simulink model "HITL_HEXA_MISSION"  (R2023b)
settings: Solver=FixedStepDiscrete  StartTime=0.0  StopTime=inf  FixedStep=1/250  RelTol=1e-3  EnableMultiTasking=on
values from neighbouring files (symbols this model uses):
  SampleTime = 1/250    (= 0.004)    [Init_FLIGHT_Hexacopter.m]    (also in Init_FLIGHT_Hexacopter_fromNCMS.m = 0.01)
undefined symbols (not defined in the file or in its folder): control, IDLEPWM, MC_PITCH_P, MC_PITCHRATE_D, MC_PITCHRATE_I, MC_PITCHRATE_P, MC_ROLL_P, MC_ROLLRATE_D, MC_ROLLRATE_I, MC_ROLLRATE_P, MC_YAW_P, MC_YAWRATE_D, MC_YAWRATE_I, MC_YAWRATE_P, MPC_XY_P, MPC_XY_VEL_MAX, MPC_Z_D, MPC_Z_I, MPC_Z_P, MPC_Z_VEL_D_ACC, MPC_Z_VEL_I_ACC, MPC_Z_VEL_MAX_DN, MPC_Z_VEL_MAX_UP, MPC_Z_VEL_P_ACC, noutputs, output, pitch, pitch_body, roll, roll_body, TargetHardware, thrust_body, timestamp, x, y, yaw, yaw_body, z
libraries: px4lib x45, px4uORBlib x19, slpidlib x10, simulink x9, px4Utilslib x5, simulink_extras x5, uavalgslib x3, px4Sensorslib x2, sharedutil x1, sharedtransform x1
(part 2 of 4)

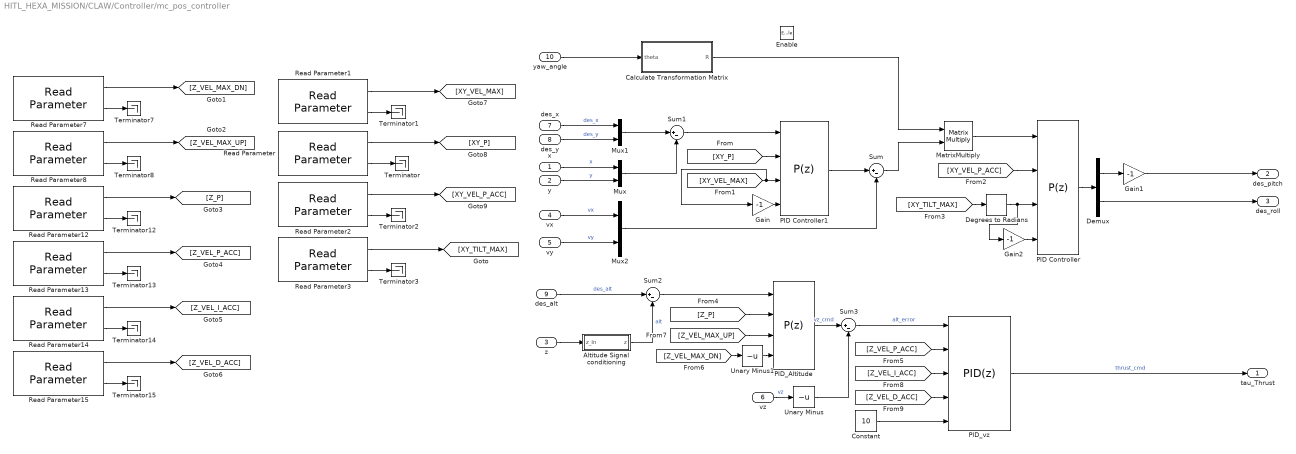
== system HITL_HEXA_MISSION/CLAW/Controller/mc_pos_controller ==
  x : Inport
  y : Inport  Port=2
  z : Inport  Port=3
  vx : Inport  Port=4
  vy : Inport  Port=5
  vz : Inport  Port=6
  des_x : Inport  Port=7
  des_y : Inport  Port=8
  des_alt : Inport  Port=9
  yaw_angle : Inport  Port=10
  Enable : EnablePort
  Altitude Signal conditioning : Subsystem
  Calculate Transformation Matrix : Subsystem
  Constant : Constant  Value=10
  Degrees to Radians : simulink_extras/Transformations/Degrees to Radians
  Demux : Demux  Outputs=2
  Gain : Gain  Gain=-1
  Gain1 : Gain  Gain=-1
  Gain2 : Gain  Gain=-1
  MatrixMultiply : Product  Multiplication=Matrix(*)
  Mux : Mux  Inputs=2
  Mux1 : Mux  Inputs=2
  Mux2 : Mux  Inputs=2
  PID Controller : slpidlib/PID Controller  Controller=P  Form=Parallel  TimeDomain=Discrete-time  UseExternalTs=off  SampleTime=-1  IntegratorMethod=Forward Euler  FilterMethod=Forward Euler  ControllerParametersSource=external  P=0.3  I=0  UseKiTs=off  D=0  N=20  UseFilter=on  TunerSelectOption=Transfer Function Based (PID Tuner App)  InitialConditionSource=internal  InitialConditionForIntegrator=0  InitialConditionForFilter=0  DifferentiatorICPrevScaledInput=0  ExternalReset=none  TrackingMode=off  Kt=1  LimitOutput=on  SatLimitsSource=external  UpperSaturationLimit=20*pi/180  LowerSaturationLimit=-20*pi/180  LinearizeAsGain=on  AntiWindupMode=clamping  Kb=1  LimitIntegrator=off  UpperIntegratorSaturationLimit=inf  LowerIntegratorSaturationLimit=-inf  POutMin=[]  POutMax=[]  IOutMin=[]  IOutMax=[]  DOutMin=[]  DOutMax=[]  NOutMin=[]  NOutMax=[]  SumOutMin=[]  SumOutMax=[]  SaturationOutMin=[]  SaturationOutMax=[]  PParamMin=[]  PParamMax=[]  IParamMin=[]  IParamMax=[]  DParamMin=[]  DParamMax=[]  NParamMin=[]  NParamMax=[]  KbParamMin=[]  KbParamMax=[]  KtParamMin=[]  KtParamMax=[]  KbOutMin=[]  KbOutMax=[]  KtOutMin=[]  KtOutMax=[]  IntegratorOutMin=[]  IntegratorOutMax=[]  FilterOutMin=[]  FilterOutMax=[]  SumI1OutMin=[]  SumI1OutMax=[]  SumI2OutMin=[]  SumI2OutMax=[]  SumI3OutMin=[]  SumI3OutMax=[]  SumI4OutMin=[]  SumI4OutMax=[]  SumDOutMin=[]  SumDOutMax=[]  DifferentiatorOutMin=[]  DifferentiatorOutMax=[]  FilterDiffOutCoefMin=[]  FilterDiffOutCoefMax=[]  ReciprocalOutMin=[]  ReciprocalOutMax=[]  SumDenOutMin=[]  SumDenOutMax=[]  SumNumOutMin=[]  SumNumOutMax=[]  DivideOutMin=[]  DivideOutMax=[]  UdiffTsProdOutMin=[]  UdiffTsProdOutMax=[]  NTsProdOutMin=[]  NTsProdOutMax=[]  UintegralTsProdOutMin=[]  UintegralTsProdOutMax=[]  UngainTsProdOutMin=[]  UngainTsProdOutMax=[]  ClampingZeroOutDataTypeStr=Inherit: Inherit via back propagation  ClampingZeroOutMin=[]  ClampingZeroOutMax=[]  FilterDenConstantOutDataTypeStr=Inherit: Inherit via back propagation  FilterDenConstantOutMin=[]  FilterDenConstantOutMax=[]  PCopyOutDataTypeStr=Inherit: Inherit via back propagation  PCopyOutMin=[]  PCopyOutMax=[]  NCopyOutDataTypeStr=Inherit: Inherit via back propagation  NCopyOutMin=[]  NCopyOutMax=[]  IntegratorContinuousStateAttributes=''  IntegratorStateMustResolveToSignalObject=off  IntegratorRTWStateStorageClass=Auto  FilterContinuousStateAttributes=''  FilterStateMustResolveToSignalObject=off  FilterRTWStateStorageClass=Auto  ParallelPVariant=ExternalParameters  IdealPVariant=Disabled  IVariant=Disabled  DVariant=Disabled  IntegratorVariant=Disabled  SatVariant=External  AWVariant=Disabled  PCopyVariant=Disabled  TRVariant=Disabled  FdbkBlocksVariant=Forward  IdealPFdbkVariant=Disabled  SatFdbkVariant=Disabled  DerivativeFilterVariant=Disabled  NVariant=Disabled  NCopyVariant=Disabled_SignalSpec  FilterICVariant=Disabled  IntegratorICVariant=Disabled  ExternalResetVariant=Disabled  TRSumVariant=Passthrough  SumFdbkVariant=Disabled  SumVariant=Passthrough_P  TsampFilterVariant=InternalTs  TsampNgainVariant=Passthrough  TsampIntegralVariant=Disabled_SignalSpec  ExternalSaturationOutDataTypeStr=Inherit: Same as second input
  PID Controller1 : slpidlib/PID Controller  Controller=P  Form=Parallel  TimeDomain=Discrete-time  UseExternalTs=off  SampleTime=-1  IntegratorMethod=Forward Euler  FilterMethod=Forward Euler  ControllerParametersSource=external  P=MPC_XY_P  I=0  UseKiTs=off  D=0  N=20  UseFilter=on  TunerSelectOption=Transfer Function Based (PID Tuner App)  InitialConditionSource=internal  InitialConditionForIntegrator=0  InitialConditionForFilter=0  DifferentiatorICPrevScaledInput=0  ExternalReset=none  TrackingMode=off  Kt=1  LimitOutput=on  SatLimitsSource=external  UpperSaturationLimit=abs(MPC_XY_VEL_MAX)  LowerSaturationLimit=-abs(MPC_XY_VEL_MAX)  LinearizeAsGain=on  AntiWindupMode=clamping  Kb=1  LimitIntegrator=off  UpperIntegratorSaturationLimit=inf  LowerIntegratorSaturationLimit=-inf  POutMin=[]  POutMax=[]  IOutMin=[]  IOutMax=[]  DOutMin=[]  DOutMax=[]  NOutMin=[]  NOutMax=[]  SumOutMin=[]  SumOutMax=[]  SaturationOutMin=[]  SaturationOutMax=[]  PParamMin=[]  PParamMax=[]  IParamMin=[]  IParamMax=[]  DParamMin=[]  DParamMax=[]  NParamMin=[]  NParamMax=[]  KbParamMin=[]  KbParamMax=[]  KtParamMin=[]  KtParamMax=[]  KbOutMin=[]  KbOutMax=[]  KtOutMin=[]  KtOutMax=[]  IntegratorOutMin=[]  IntegratorOutMax=[]  FilterOutMin=[]  FilterOutMax=[]  SumI1OutMin=[]  SumI1OutMax=[]  SumI2OutMin=[]  SumI2OutMax=[]  SumI3OutMin=[]  SumI3OutMax=[]  SumI4OutMin=[]  SumI4OutMax=[]  SumDOutMin=[]  SumDOutMax=[]  DifferentiatorOutMin=[]  DifferentiatorOutMax=[]  FilterDiffOutCoefMin=[]  FilterDiffOutCoefMax=[]  ReciprocalOutMin=[]  ReciprocalOutMax=[]  SumDenOutMin=[]  SumDenOutMax=[]  SumNumOutMin=[]  SumNumOutMax=[]  DivideOutMin=[]  DivideOutMax=[]  UdiffTsProdOutMin=[]  UdiffTsProdOutMax=[]  NTsProdOutMin=[]  NTsProdOutMax=[]  UintegralTsProdOutMin=[]  UintegralTsProdOutMax=[]  UngainTsProdOutMin=[]  UngainTsProdOutMax=[]  ClampingZeroOutDataTypeStr=Inherit: Inherit via back propagation  ClampingZeroOutMin=[]  ClampingZeroOutMax=[]  FilterDenConstantOutDataTypeStr=Inherit: Inherit via back propagation  FilterDenConstantOutMin=[]  FilterDenConstantOutMax=[]  PCopyOutDataTypeStr=Inherit: Inherit via back propagation  PCopyOutMin=[]  PCopyOutMax=[]  NCopyOutDataTypeStr=Inherit: Inherit via back propagation  NCopyOutMin=[]  NCopyOutMax=[]  IntegratorContinuousStateAttributes=''  IntegratorStateMustResolveToSignalObject=off  IntegratorRTWStateStorageClass=Auto  FilterContinuousStateAttributes=''  FilterStateMustResolveToSignalObject=off  FilterRTWStateStorageClass=Auto  ParallelPVariant=ExternalParameters  IdealPVariant=Disabled  IVariant=Disabled  DVariant=Disabled  IntegratorVariant=Disabled  SatVariant=External  AWVariant=Disabled  PCopyVariant=Disabled  TRVariant=Disabled  FdbkBlocksVariant=Forward  IdealPFdbkVariant=Disabled  SatFdbkVariant=Disabled  DerivativeFilterVariant=Disabled  NVariant=Disabled  NCopyVariant=Disabled_SignalSpec  FilterICVariant=Disabled  IntegratorICVariant=Disabled  ExternalResetVariant=Disabled  TRSumVariant=Passthrough  SumFdbkVariant=Disabled  SumVariant=Passthrough_P  TsampFilterVariant=InternalTs  TsampNgainVariant=Passthrough  TsampIntegralVariant=Disabled_SignalSpec  ExternalSaturationOutDataTypeStr=Inherit: Same as second input
  PID_Altitude : slpidlib/PID Controller  Controller=P  Form=Parallel  TimeDomain=Discrete-time  UseExternalTs=off  SampleTime=-1  IntegratorMethod=Backward Euler  FilterMethod=Forward Euler  ControllerParametersSource=external  P=MPC_Z_P  I=MPC_Z_I  UseKiTs=off  D=MPC_Z_D  N=10  UseFilter=on  TunerSelectOption=Transfer Function Based (PID Tuner App)  InitialConditionSource=internal  InitialConditionForIntegrator=0  InitialConditionForFilter=0  DifferentiatorICPrevScaledInput=0  ExternalReset=none  TrackingMode=off  Kt=1  LimitOutput=on  SatLimitsSource=external  UpperSaturationLimit=MPC_Z_VEL_MAX_UP  LowerSaturationLimit=-abs(MPC_Z_VEL_MAX_DN)  LinearizeAsGain=off  AntiWindupMode=clamping  Kb=1  LimitIntegrator=off  UpperIntegratorSaturationLimit=inf  LowerIntegratorSaturationLimit=-inf  POutMin=[]  POutMax=[]  IOutMin=[]  IOutMax=[]  DOutMin=[]  DOutMax=[]  NOutMin=[]  NOutMax=[]  SumOutMin=[]  SumOutMax=[]  SaturationOutMin=[]  SaturationOutMax=[]  PParamMin=[]  PParamMax=[]  IParamMin=[]  IParamMax=[]  DParamMin=[]  DParamMax=[]  NParamMin=[]  NParamMax=[]  KbParamMin=[]  KbParamMax=[]  KtParamMin=[]  KtParamMax=[]  KbOutMin=[]  KbOutMax=[]  KtOutMin=[]  KtOutMax=[]  IntegratorOutMin=[]  IntegratorOutMax=[]  FilterOutMin=[]  FilterOutMax=[]  SumI1OutMin=[]  SumI1OutMax=[]  SumI2OutMin=[]  SumI2OutMax=[]  SumI3OutMin=[]  SumI3OutMax=[]  SumI4OutMin=[]  SumI4OutMax=[]  SumDOutMin=[]  SumDOutMax=[]  DifferentiatorOutMin=[]  DifferentiatorOutMax=[]  FilterDiffOutCoefMin=[]  FilterDiffOutCoefMax=[]  ReciprocalOutMin=[]  ReciprocalOutMax=[]  SumDenOutMin=[]  SumDenOutMax=[]  SumNumOutMin=[]  SumNumOutMax=[]  DivideOutMin=[]  DivideOutMax=[]  UdiffTsProdOutMin=[]  UdiffTsProdOutMax=[]  NTsProdOutMin=[]  NTsProdOutMax=[]  UintegralTsProdOutMin=[]  UintegralTsProdOutMax=[]  UngainTsProdOutMin=[]  UngainTsProdOutMax=[]  ClampingZeroOutDataTypeStr=Inherit: Inherit via back propagation  ClampingZeroOutMin=[]  ClampingZeroOutMax=[]  FilterDenConstantOutDataTypeStr=Inherit: Inherit via back propagation  FilterDenConstantOutMin=[]  FilterDenConstantOutMax=[]  PCopyOutDataTypeStr=Inherit: Inherit via back propagation  PCopyOutMin=[]  PCopyOutMax=[]  NCopyOutDataTypeStr=Inherit: Inherit via back propagation  NCopyOutMin=[]  NCopyOutMax=[]  IntegratorContinuousStateAttributes=''  IntegratorStateMustResolveToSignalObject=off  IntegratorRTWStateStorageClass=Auto  FilterContinuousStateAttributes=''  FilterStateMustResolveToSignalObject=off  FilterRTWStateStorageClass=Auto  ParallelPVariant=ExternalParameters  IdealPVariant=Disabled  IVariant=Disabled  DVariant=Disabled  IntegratorVariant=Disabled  SatVariant=External  AWVariant=Disabled  PCopyVariant=Disabled  TRVariant=Disabled  FdbkBlocksVariant=Forward  IdealPFdbkVariant=Disabled  SatFdbkVariant=Disabled  DerivativeFilterVariant=Disabled  NVariant=Disabled  NCopyVariant=Disabled_SignalSpec  FilterICVariant=Disabled  IntegratorICVariant=Disabled  ExternalResetVariant=Disabled  TRSumVariant=Passthrough  SumFdbkVariant=Disabled  SumVariant=Passthrough_P  TsampFilterVariant=InternalTs  TsampNgainVariant=Passthrough  TsampIntegralVariant=Disabled_SignalSpec  ExternalSaturationOutDataTypeStr=Inherit: Same as second input
  PID_vz : slpidlib/PID Controller  Controller=PID  Form=Parallel  TimeDomain=Discrete-time  UseExternalTs=off  SampleTime=-1  IntegratorMethod=Backward Euler  FilterMethod=Forward Euler  ControllerParametersSource=external  P=MPC_Z_VEL_P_ACC  I=MPC_Z_VEL_I_ACC  UseKiTs=off  D=MPC_Z_VEL_D_ACC  N=10  UseFilter=on  TunerSelectOption=Transfer Function Based (PID Tuner App)  InitialConditionSource=internal  InitialConditionForIntegrator=0  InitialConditionForFilter=0  DifferentiatorICPrevScaledInput=0  ExternalReset=none  TrackingMode=off  Kt=1  LimitOutput=on  SatLimitsSource=internal  UpperSaturationLimit=1  LowerSaturationLimit=0  LinearizeAsGain=off  AntiWindupMode=clamping  Kb=1  LimitIntegrator=off  UpperIntegratorSaturationLimit=inf  LowerIntegratorSaturationLimit=-inf  POutMin=[]  POutMax=[]  IOutMin=[]  IOutMax=[]  DOutMin=[]  DOutMax=[]  NOutMin=[]  NOutMax=[]  SumOutMin=[]  SumOutMax=[]  SaturationOutMin=[]  SaturationOutMax=[]  PParamMin=[]  PParamMax=[]  IParamMin=[]  IParamMax=[]  DParamMin=[]  DParamMax=[]  NParamMin=[]  NParamMax=[]  KbParamMin=[]  KbParamMax=[]  KtParamMin=[]  KtParamMax=[]  KbOutMin=[]  KbOutMax=[]  KtOutMin=[]  KtOutMax=[]  IntegratorOutMin=[]  IntegratorOutMax=[]  FilterOutMin=[]  FilterOutMax=[]  SumI1OutMin=[]  SumI1OutMax=[]  SumI2OutMin=[]  SumI2OutMax=[]  SumI3OutMin=[]  SumI3OutMax=[]  SumI4OutMin=[]  SumI4OutMax=[]  SumDOutMin=[]  SumDOutMax=[]  DifferentiatorOutMin=[]  DifferentiatorOutMax=[]  FilterDiffOutCoefMin=[]  FilterDiffOutCoefMax=[]  ReciprocalOutMin=[]  ReciprocalOutMax=[]  SumDenOutMin=[]  SumDenOutMax=[]  SumNumOutMin=[]  SumNumOutMax=[]  DivideOutMin=[]  DivideOutMax=[]  UdiffTsProdOutMin=[]  UdiffTsProdOutMax=[]  NTsProdOutMin=[]  NTsProdOutMax=[]  UintegralTsProdOutMin=[]  UintegralTsProdOutMax=[]  UngainTsProdOutMin=[]  UngainTsProdOutMax=[]  ClampingZeroOutDataTypeStr=Inherit: Inherit via back propagation  ClampingZeroOutMin=[]  ClampingZeroOutMax=[]  FilterDenConstantOutDataTypeStr=Inherit: Inherit via back propagation  FilterDenConstantOutMin=[]  FilterDenConstantOutMax=[]  PCopyOutDataTypeStr=Inherit: Inherit via back propagation  PCopyOutMin=[]  PCopyOutMax=[]  NCopyOutDataTypeStr=Inherit: Inherit via back propagation  NCopyOutMin=[]  NCopyOutMax=[]  IntegratorContinuousStateAttributes=''  IntegratorStateMustResolveToSignalObject=off  IntegratorRTWStateStorageClass=Auto  FilterContinuousStateAttributes=''  FilterStateMustResolveToSignalObject=off  FilterRTWStateStorageClass=Auto  ParallelPVariant=ExternalParameters  IdealPVariant=Disabled  IVariant=ExternalParameters  DVariant=ExternalParameters  IntegratorVariant=Discrete  SatVariant=Enabled  AWVariant=DiscClampingParallel  PCopyVariant=Disabled  TRVariant=Disabled  FdbkBlocksVariant=Feedback  IdealPFdbkVariant=Passthrough  SatFdbkVariant=Passthrough  DerivativeFilterVariant=ForwardEulerFilter  NVariant=ExternalParameters  NCopyVariant=Disabled  FilterICVariant=InternalICsFilter  IntegratorICVariant=InternalICs  ExternalResetVariant=Disabled  TRSumVariant=Passthrough  SumFdbkVariant=Enabled  SumVariant=Sum_PID  TsampFilterVariant=InternalTs  TsampNgainVariant=Passthrough  TsampIntegralVariant=Disabled_SignalSpec  ExternalSaturationOutDataTypeStr=Inherit: Same as second input
  Read Parameter : px4lib/Read Parameter  ParameterName=SL_XY_P  DataType=FLOAT  SampleTime=-1
  Read Parameter1 : px4lib/Read Parameter  ParameterName=SL_XY_VEL_MAX  DataType=FLOAT  SampleTime=-1
  Read Parameter12 : px4lib/Read Parameter  ParameterName=SL_Z_P  DataType=FLOAT  SampleTime=-1
  Read Parameter13 : px4lib/Read Parameter  ParameterName=SL_Z_VEL_P_ACC  DataType=FLOAT  SampleTime=-1
  Read Parameter14 : px4lib/Read Parameter  ParameterName=SL_Z_VEL_I_ACC  DataType=FLOAT  SampleTime=-1
  Read Parameter15 : px4lib/Read Parameter  ParameterName=SL_Z_VEL_D_ACC  DataType=FLOAT  SampleTime=-1
  Read Parameter2 : px4lib/Read Parameter  ParameterName=SL_XY_VEL_P_ACC  DataType=FLOAT  SampleTime=-1
  Read Parameter3 : px4lib/Read Parameter  ParameterName=SL_XY_TILT_MAX  DataType=FLOAT  SampleTime=-1
  Read Parameter7 : px4lib/Read Parameter  ParameterName=SL_Z_VEL_MAX_DN  DataType=FLOAT  SampleTime=-1
  Read Parameter8 : px4lib/Read Parameter  ParameterName=SL_Z_VEL_MAX_UP  DataType=FLOAT  SampleTime=-1
  Sum{,1..3} (4 alike) : Sum  Inputs=|+-
  Terminator{,1..3,7..8,12..15} (10 alike) : Terminator
  Unary Minus : UnaryMinus
  Unary Minus1 : UnaryMinus
  tau_Thrust : Outport
  des_pitch : Outport  Port=2
  des_roll : Outport  Port=3
  wires:
  des_alt/1 -> Sum2/1  "des_alt"
  Calculate Transformation Matrix/1(R) -> MatrixMultiply/1
  yaw_angle/1 -> Calculate Transformation Matrix/1(theta)
  Altitude Signal conditioning/1(z) -> Sum2/2  "alt"
  PID_Altitude/1 -> Sum3/1  "vz_cmd"
  vz/1 -> Unary Minus/1  "vz"
  PID_vz/1 -> tau_Thrust/1  "thrust_cmd"
  vx/1 -> Mux2/1  "vx"
  vy/1 -> Mux2/2  "vy"
  Sum2/1 -> PID_Altitude/1
  z/1 -> Altitude Signal conditioning/1(z_In)
  PID Controller/1 -> Demux/1
  Demux/1 -> Gain1/1
  x/1 -> Mux/1  "x"
  y/1 -> Mux/2  "y"
  Demux/2 -> des_roll/1
  Sum/1 -> MatrixMultiply/2
  Mux/1 -> Sum1/2
  Sum1/1 -> PID Controller1/1
  Unary Minus/1 -> Sum3/2
  Sum3/1 -> PID_vz/1  "alt_error"
  des_x/1 -> Mux1/1  "des_x"
  des_y/1 -> Mux1/2  "des_y"
  MatrixMultiply/1 -> PID Controller/1
  PID Controller1/1 -> Sum/1
  Mux1/1 -> Sum1/1
  Gain1/1 -> des_pitch/1
  Mux2/1 -> Sum/2
  Read Parameter14/2 -> Terminator14/1
  Read Parameter12/2 -> Terminator12/1
  Read Parameter14/1 -> [Z_VEL_I_ACC]
  Read Parameter/1 -> [XY_P]
  Read Parameter13/1 -> [Z_VEL_P_ACC]
  Read Parameter8/1 -> [Z_VEL_MAX_UP]
  Read Parameter3/2 -> Terminator3/1
  Read Parameter12/1 -> [Z_P]
  Read Parameter8/2 -> Terminator8/1
  Read Parameter7/2 -> Terminator7/1
  Read Parameter1/1 -> [XY_VEL_MAX]
  Read Parameter2/1 -> [XY_VEL_P_ACC]
  Read Parameter2/2 -> Terminator2/1
  Read Parameter15/1 -> [Z_VEL_D_ACC]
  Read Parameter1/2 -> Terminator1/1
  Read Parameter3/1 -> [XY_TILT_MAX]
  Read Parameter13/2 -> Terminator13/1
  Read Parameter/2 -> Terminator/1
  Read Parameter15/2 -> Terminator15/1
  [XY_P] -> PID Controller1/2
  [XY_VEL_MAX] -> PID Controller1/3, Gain/1
  Gain/1 -> PID Controller1/4
  [XY_VEL_P_ACC] -> PID Controller/2
  [XY_TILT_MAX] -> Degrees to Radians/1
  Degrees to Radians/1 -> Gain2/1, PID Controller/3
  Gain2/1 -> PID Controller/4
  Read Parameter7/1 -> [Z_VEL_MAX_DN]
  [Z_P] -> PID_Altitude/2
  [Z_VEL_MAX_UP] -> PID_Altitude/3
  [Z_VEL_P_ACC] -> PID_vz/2
  [Z_VEL_I_ACC] -> PID_vz/3
  [Z_VEL_D_ACC] -> PID_vz/4
  Constant/1 -> PID_vz/5
  [Z_VEL_MAX_DN] -> Unary Minus1/1
  Unary Minus1/1 -> PID_Altitude/4

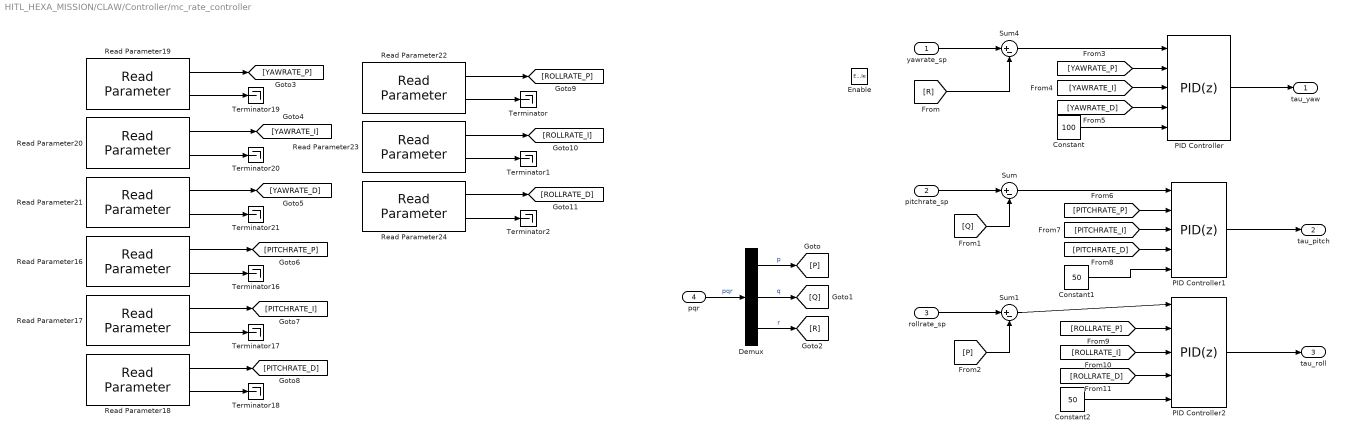
== system HITL_HEXA_MISSION/CLAW/Controller/mc_rate_controller ==
  yawrate_sp : Inport
  pitchrate_sp : Inport  Port=2
  rollrate_sp : Inport  Port=3
  pqr : Inport  Port=4
  Enable : EnablePort
  Constant : Constant  Value=100
  Constant1 : Constant  Value=50
  Constant2 : Constant  Value=50
  Demux : Demux  Outputs=3
  PID Controller : slpidlib/PID Controller  Controller=PID  Form=Parallel  TimeDomain=Discrete-time  UseExternalTs=off  SampleTime=-1  IntegratorMethod=Forward Euler  FilterMethod=Forward Euler  ControllerParametersSource=external  P=MC_YAWRATE_P  I=MC_YAWRATE_I  UseKiTs=off  D=MC_YAWRATE_D  N=100  UseFilter=on  TunerSelectOption=Transfer Function Based (PID Tuner App)  InitialConditionSource=internal  InitialConditionForIntegrator=0  InitialConditionForFilter=0  DifferentiatorICPrevScaledInput=0  ExternalReset=none  TrackingMode=off  Kt=1  LimitOutput=on  SatLimitsSource=internal  UpperSaturationLimit=0.1  LowerSaturationLimit=-0.1  LinearizeAsGain=on  AntiWindupMode=clamping  Kb=1  LimitIntegrator=off  UpperIntegratorSaturationLimit=inf  LowerIntegratorSaturationLimit=-inf  POutMin=[]  POutMax=[]  IOutMin=[]  IOutMax=[]  DOutMin=[]  DOutMax=[]  NOutMin=[]  NOutMax=[]  SumOutMin=[]  SumOutMax=[]  SaturationOutMin=[]  SaturationOutMax=[]  PParamMin=[]  PParamMax=[]  IParamMin=[]  IParamMax=[]  DParamMin=[]  DParamMax=[]  NParamMin=[]  NParamMax=[]  KbParamMin=[]  KbParamMax=[]  KtParamMin=[]  KtParamMax=[]  KbOutMin=[]  KbOutMax=[]  KtOutMin=[]  KtOutMax=[]  IntegratorOutMin=[]  IntegratorOutMax=[]  FilterOutMin=[]  FilterOutMax=[]  SumI1OutMin=[]  SumI1OutMax=[]  SumI2OutMin=[]  SumI2OutMax=[]  SumI3OutMin=[]  SumI3OutMax=[]  SumI4OutMin=[]  SumI4OutMax=[]  SumDOutMin=[]  SumDOutMax=[]  DifferentiatorOutMin=[]  DifferentiatorOutMax=[]  FilterDiffOutCoefMin=[]  FilterDiffOutCoefMax=[]  ReciprocalOutMin=[]  ReciprocalOutMax=[]  SumDenOutMin=[]  SumDenOutMax=[]  SumNumOutMin=[]  SumNumOutMax=[]  DivideOutMin=[]  DivideOutMax=[]  UdiffTsProdOutMin=[]  UdiffTsProdOutMax=[]  NTsProdOutMin=[]  NTsProdOutMax=[]  UintegralTsProdOutMin=[]  UintegralTsProdOutMax=[]  UngainTsProdOutMin=[]  UngainTsProdOutMax=[]  ClampingZeroOutDataTypeStr=Inherit: Inherit via back propagation  ClampingZeroOutMin=[]  ClampingZeroOutMax=[]  FilterDenConstantOutDataTypeStr=Inherit: Inherit via back propagation  FilterDenConstantOutMin=[]  FilterDenConstantOutMax=[]  PCopyOutDataTypeStr=Inherit: Inherit via back propagation  PCopyOutMin=[]  PCopyOutMax=[]  NCopyOutDataTypeStr=Inherit: Inherit via back propagation  NCopyOutMin=[]  NCopyOutMax=[]  IntegratorContinuousStateAttributes=''  IntegratorStateMustResolveToSignalObject=off  IntegratorRTWStateStorageClass=Auto  FilterContinuousStateAttributes=''  FilterStateMustResolveToSignalObject=off  FilterRTWStateStorageClass=Auto  ParallelPVariant=ExternalParameters  IdealPVariant=Disabled  IVariant=ExternalParameters  DVariant=ExternalParameters  IntegratorVariant=Discrete  SatVariant=Enabled  AWVariant=DiscClampingParallel  PCopyVariant=Disabled  TRVariant=Disabled  FdbkBlocksVariant=Forward  IdealPFdbkVariant=Disabled  SatFdbkVariant=Disabled  DerivativeFilterVariant=ForwardEulerFilter  NVariant=ExternalParameters  NCopyVariant=Disabled  FilterICVariant=InternalICsFilter  IntegratorICVariant=InternalICs  ExternalResetVariant=Disabled  TRSumVariant=Passthrough  SumFdbkVariant=Disabled  SumVariant=Sum_PID  TsampFilterVariant=InternalTs  TsampNgainVariant=Passthrough  TsampIntegralVariant=Disabled_SignalSpec  ExternalSaturationOutDataTypeStr=Inherit: Same as second input
  PID Controller1 : slpidlib/PID Controller  Controller=PID  Form=Parallel  TimeDomain=Discrete-time  UseExternalTs=off  SampleTime=-1  IntegratorMethod=Forward Euler  FilterMethod=Forward Euler  ControllerParametersSource=external  P=MC_PITCHRATE_P  I=MC_PITCHRATE_I  UseKiTs=off  D=MC_PITCHRATE_D  N=50  UseFilter=on  TunerSelectOption=Transfer Function Based (PID Tuner App)  InitialConditionSource=internal  InitialConditionForIntegrator=0  InitialConditionForFilter=0  DifferentiatorICPrevScaledInput=0  ExternalReset=none  TrackingMode=off  Kt=1  LimitOutput=on  SatLimitsSource=internal  UpperSaturationLimit=0.2  LowerSaturationLimit=-0.2  LinearizeAsGain=on  AntiWindupMode=clamping  Kb=1  LimitIntegrator=off  UpperIntegratorSaturationLimit=inf  LowerIntegratorSaturationLimit=-inf  POutMin=[]  POutMax=[]  IOutMin=[]  IOutMax=[]  DOutMin=[]  DOutMax=[]  NOutMin=[]  NOutMax=[]  SumOutMin=[]  SumOutMax=[]  SaturationOutMin=[]  SaturationOutMax=[]  PParamMin=[]  PParamMax=[]  IParamMin=[]  IParamMax=[]  DParamMin=[]  DParamMax=[]  NParamMin=[]  NParamMax=[]  KbParamMin=[]  KbParamMax=[]  KtParamMin=[]  KtParamMax=[]  KbOutMin=[]  KbOutMax=[]  KtOutMin=[]  KtOutMax=[]  IntegratorOutMin=[]  IntegratorOutMax=[]  FilterOutMin=[]  FilterOutMax=[]  SumI1OutMin=[]  SumI1OutMax=[]  SumI2OutMin=[]  SumI2OutMax=[]  SumI3OutMin=[]  SumI3OutMax=[]  SumI4OutMin=[]  SumI4OutMax=[]  SumDOutMin=[]  SumDOutMax=[]  DifferentiatorOutMin=[]  DifferentiatorOutMax=[]  FilterDiffOutCoefMin=[]  FilterDiffOutCoefMax=[]  ReciprocalOutMin=[]  ReciprocalOutMax=[]  SumDenOutMin=[]  SumDenOutMax=[]  SumNumOutMin=[]  SumNumOutMax=[]  DivideOutMin=[]  DivideOutMax=[]  UdiffTsProdOutMin=[]  UdiffTsProdOutMax=[]  NTsProdOutMin=[]  NTsProdOutMax=[]  UintegralTsProdOutMin=[]  UintegralTsProdOutMax=[]  UngainTsProdOutMin=[]  UngainTsProdOutMax=[]  ClampingZeroOutDataTypeStr=Inherit: Inherit via back propagation  ClampingZeroOutMin=[]  ClampingZeroOutMax=[]  FilterDenConstantOutDataTypeStr=Inherit: Inherit via back propagation  FilterDenConstantOutMin=[]  FilterDenConstantOutMax=[]  PCopyOutDataTypeStr=Inherit: Inherit via back propagation  PCopyOutMin=[]  PCopyOutMax=[]  NCopyOutDataTypeStr=Inherit: Inherit via back propagation  NCopyOutMin=[]  NCopyOutMax=[]  IntegratorContinuousStateAttributes=''  IntegratorStateMustResolveToSignalObject=off  IntegratorRTWStateStorageClass=Auto  FilterContinuousStateAttributes=''  FilterStateMustResolveToSignalObject=off  FilterRTWStateStorageClass=Auto  ParallelPVariant=ExternalParameters  IdealPVariant=Disabled  IVariant=ExternalParameters  DVariant=ExternalParameters  IntegratorVariant=Discrete  SatVariant=Enabled  AWVariant=DiscClampingParallel  PCopyVariant=Disabled  TRVariant=Disabled  FdbkBlocksVariant=Forward  IdealPFdbkVariant=Disabled  SatFdbkVariant=Disabled  DerivativeFilterVariant=ForwardEulerFilter  NVariant=ExternalParameters  NCopyVariant=Disabled  FilterICVariant=InternalICsFilter  IntegratorICVariant=InternalICs  ExternalResetVariant=Disabled  TRSumVariant=Passthrough  SumFdbkVariant=Disabled  SumVariant=Sum_PID  TsampFilterVariant=InternalTs  TsampNgainVariant=Passthrough  TsampIntegralVariant=Disabled_SignalSpec  ExternalSaturationOutDataTypeStr=Inherit: Same as second input
  PID Controller2 : slpidlib/PID Controller  Controller=PID  Form=Parallel  TimeDomain=Discrete-time  UseExternalTs=off  SampleTime=-1  IntegratorMethod=Forward Euler  FilterMethod=Forward Euler  ControllerParametersSource=external  P=MC_ROLLRATE_P  I=MC_ROLLRATE_I  UseKiTs=off  D=MC_ROLLRATE_D  N=50  UseFilter=on  TunerSelectOption=Transfer Function Based (PID Tuner App)  InitialConditionSource=internal  InitialConditionForIntegrator=0  InitialConditionForFilter=0  DifferentiatorICPrevScaledInput=0  ExternalReset=none  TrackingMode=off  Kt=1  LimitOutput=on  SatLimitsSource=internal  UpperSaturationLimit=0.2  LowerSaturationLimit=-0.2  LinearizeAsGain=on  AntiWindupMode=clamping  Kb=1  LimitIntegrator=off  UpperIntegratorSaturationLimit=inf  LowerIntegratorSaturationLimit=-inf  POutMin=[]  POutMax=[]  IOutMin=[]  IOutMax=[]  DOutMin=[]  DOutMax=[]  NOutMin=[]  NOutMax=[]  SumOutMin=[]  SumOutMax=[]  SaturationOutMin=[]  SaturationOutMax=[]  PParamMin=[]  PParamMax=[]  IParamMin=[]  IParamMax=[]  DParamMin=[]  DParamMax=[]  NParamMin=[]  NParamMax=[]  KbParamMin=[]  KbParamMax=[]  KtParamMin=[]  KtParamMax=[]  KbOutMin=[]  KbOutMax=[]  KtOutMin=[]  KtOutMax=[]  IntegratorOutMin=[]  IntegratorOutMax=[]  FilterOutMin=[]  FilterOutMax=[]  SumI1OutMin=[]  SumI1OutMax=[]  SumI2OutMin=[]  SumI2OutMax=[]  SumI3OutMin=[]  SumI3OutMax=[]  SumI4OutMin=[]  SumI4OutMax=[]  SumDOutMin=[]  SumDOutMax=[]  DifferentiatorOutMin=[]  DifferentiatorOutMax=[]  FilterDiffOutCoefMin=[]  FilterDiffOutCoefMax=[]  ReciprocalOutMin=[]  ReciprocalOutMax=[]  SumDenOutMin=[]  SumDenOutMax=[]  SumNumOutMin=[]  SumNumOutMax=[]  DivideOutMin=[]  DivideOutMax=[]  UdiffTsProdOutMin=[]  UdiffTsProdOutMax=[]  NTsProdOutMin=[]  NTsProdOutMax=[]  UintegralTsProdOutMin=[]  UintegralTsProdOutMax=[]  UngainTsProdOutMin=[]  UngainTsProdOutMax=[]  ClampingZeroOutDataTypeStr=Inherit: Inherit via back propagation  ClampingZeroOutMin=[]  ClampingZeroOutMax=[]  FilterDenConstantOutDataTypeStr=Inherit: Inherit via back propagation  FilterDenConstantOutMin=[]  FilterDenConstantOutMax=[]  PCopyOutDataTypeStr=Inherit: Inherit via back propagation  PCopyOutMin=[]  PCopyOutMax=[]  NCopyOutDataTypeStr=Inherit: Inherit via back propagation  NCopyOutMin=[]  NCopyOutMax=[]  IntegratorContinuousStateAttributes=''  IntegratorStateMustResolveToSignalObject=off  IntegratorRTWStateStorageClass=Auto  FilterContinuousStateAttributes=''  FilterStateMustResolveToSignalObject=off  FilterRTWStateStorageClass=Auto  ParallelPVariant=ExternalParameters  IdealPVariant=Disabled  IVariant=ExternalParameters  DVariant=ExternalParameters  IntegratorVariant=Discrete  SatVariant=Enabled  AWVariant=DiscClampingParallel  PCopyVariant=Disabled  TRVariant=Disabled  FdbkBlocksVariant=Forward  IdealPFdbkVariant=Disabled  SatFdbkVariant=Disabled  DerivativeFilterVariant=ForwardEulerFilter  NVariant=ExternalParameters  NCopyVariant=Disabled  FilterICVariant=InternalICsFilter  IntegratorICVariant=InternalICs  ExternalResetVariant=Disabled  TRSumVariant=Passthrough  SumFdbkVariant=Disabled  SumVariant=Sum_PID  TsampFilterVariant=InternalTs  TsampNgainVariant=Passthrough  TsampIntegralVariant=Disabled_SignalSpec  ExternalSaturationOutDataTypeStr=Inherit: Same as second input
  Read Parameter16 : px4lib/Read Parameter  ParameterName=SL_PITCHRATE_P  DataType=FLOAT  SampleTime=-1
  Read Parameter17 : px4lib/Read Parameter  ParameterName=SL_PITCHRATE_I  DataType=FLOAT  SampleTime=-1
  Read Parameter18 : px4lib/Read Parameter  ParameterName=SL_PITCHRATE_D  DataType=FLOAT  SampleTime=-1
  Read Parameter19 : px4lib/Read Parameter  ParameterName=SL_YAWRATE_P  DataType=FLOAT  SampleTime=-1
  Read Parameter20 : px4lib/Read Parameter  ParameterName=SL_YAWRATE_I  DataType=FLOAT  SampleTime=-1
  Read Parameter21 : px4lib/Read Parameter  ParameterName=SL_YAWRATE_D  DataType=FLOAT  SampleTime=-1
  Read Parameter22 : px4lib/Read Parameter  ParameterName=SL_ROLLRATE_P  DataType=FLOAT  SampleTime=-1
  Read Parameter23 : px4lib/Read Parameter  ParameterName=SL_ROLLRATE_I  DataType=FLOAT  SampleTime=-1
  Read Parameter24 : px4lib/Read Parameter  ParameterName=SL_ROLLRATE_D  DataType=FLOAT  SampleTime=-1
  Sum : Sum  Inputs=|+-
  Sum1 : Sum  Inputs=|+-
  Sum4 : Sum  Inputs=|+-
  Terminator{,1..2,16..21} (9 alike) : Terminator
  tau_yaw : Outport
  tau_pitch : Outport  Port=2
  tau_roll : Outport  Port=3
  wires:
  PID Controller2/1 -> tau_roll/1
  Sum4/1 -> PID Controller/1
  PID Controller1/1 -> tau_pitch/1
  Sum1/1 -> PID Controller2/1
  PID Controller/1 -> tau_yaw/1
  Sum/1 -> PID Controller1/1
  pqr/1 -> Demux/1  "pqr"
  pitchrate_sp/1 -> Sum/1
  rollrate_sp/1 -> Sum1/1
  yawrate_sp/1 -> Sum4/1
  Demux/1 -> [P]  "p"
  Demux/2 -> [Q]  "q"
  Demux/3 -> [R]  "r"
  [R] -> Sum4/2
  [Q] -> Sum/2
  [P] -> Sum1/2
  Read Parameter22/1 -> [ROLLRATE_P]
  Read Parameter20/2 -> Terminator20/1
  Read Parameter17/1 -> [PITCHRATE_I]
  Read Parameter21/2 -> Terminator21/1
  Read Parameter19/1 -> [YAWRATE_P]
  Read Parameter18/2 -> Terminator18/1
  Read Parameter17/2 -> Terminator17/1
  Read Parameter16/1 -> [PITCHRATE_P]
  Read Parameter16/2 -> Terminator16/1
  Read Parameter24/2 -> Terminator2/1
  Read Parameter23/2 -> Terminator1/1
  Read Parameter18/1 -> [PITCHRATE_D]
  Read Parameter19/2 -> Terminator19/1
  Read Parameter22/2 -> Terminator/1
  Read Parameter23/1 -> [ROLLRATE_I]
  Read Parameter20/1 -> [YAWRATE_I]
  Read Parameter21/1 -> [YAWRATE_D]
  Read Parameter24/1 -> [ROLLRATE_D]
  [YAWRATE_P] -> PID Controller/2
  [YAWRATE_I] -> PID Controller/3
  [YAWRATE_D] -> PID Controller/4
  Constant/1 -> PID Controller/5
  [PITCHRATE_P] -> PID Controller1/2
  [PITCHRATE_I] -> PID Controller1/3
  [PITCHRATE_D] -> PID Controller1/4
  Constant1/1 -> PID Controller1/5
  [ROLLRATE_P] -> PID Controller2/2
  [ROLLRATE_I] -> PID Controller2/3
  [ROLLRATE_D] -> PID Controller2/4
  Constant2/1 -> PID Controller2/5

== system HITL_HEXA_MISSION/CLAW/Controller/readParameters ==
  Terminator{4..5,22..24} (5 alike) : Terminator
  Bus Element Out22 : Outport  PortName=param  Element=ROLLRATE_I
  Bus Element Out23 : Outport  PortName=param  Element=ROLLRATE_D
  Bus Element Out24 : Outport  PortName=param  Element=ROLLRATE_P
  wires:
  ? -> Terminator5/1
  ? -> Terminator4/1
  ? -> ?

== system HITL_HEXA_MISSION/Navigation/Quadcopter Navigation Algorithm/Manual Waypoints ==
  Current Position : Inport
  Constant1 : Constant  Value=[0 0 -20 0; 20 0 -20 0;20 10 -20 0; 20 100 -30 0;30 100 -30 0;50 100 -30 0]  SampleTime=-1
  Constant2 : Constant  Value=2  SampleTime=-1
  Constant3 : Constant  Value=0  SampleTime=-1
  Mux : Mux  Inputs=2
  Subsystem : Subsystem
  Switch : Switch  Criteria=u2 > Threshold  SaturateOnIntegerOverflow=off  InputSameDT=off
  Terminator1 : Terminator
  Terminator2 : Terminator
  Terminator4 : Terminator
  Waypoint Follower : uavalgslib/Waypoint Follower  UAVType=multirotor  StartFrom=first  TransitionRadiusSource=internal  TransitionRadius=5  MinLookaheadDistance=0.1  YawInput=on  ShowCrossTrackErrorOutput=off  ShowStatusOutput=on  SimulateUsing=Interpreted execution
  Desired Position : Outport
  wires:
  Constant1/1 -> Waypoint Follower/2
  Waypoint Follower/1 -> Subsystem/2(Lookahead Point), Switch/3
  Waypoint Follower/4 -> Terminator4/1
  Subsystem/1(des_landing_pos) -> Switch/1
  Current Position/1 -> Waypoint Follower/1, Subsystem/1(curr_xyzYaw)
  Waypoint Follower/5 -> Switch/2
  Constant2/1 -> Waypoint Follower/3
  Waypoint Follower/2 -> Terminator2/1
  Switch/1 -> Mux/1  "command"
  Mux/1 -> Desired Position/1
  Waypoint Follower/3 -> Terminator1/1
  Constant3/1 -> Mux/2

== system HITL_HEXA_MISSION/Navigation/Quadcopter Navigation Algorithm/Manual Waypoints from Simulink Dashboard ==
  note: Desired XY Position, Altitude and Yaw can be changed by these sliders
  Current Position : Inport  PortDimensions=[1 4]
  Degrees to Radians : simulink_extras/Transformations/Degrees to Radians
  Gain : Gain  Gain=-1
  Manual Switch : ManualSwitch
  Manual Switch1 : ManualSwitch
  Mux : Mux
  Sine Wave : Sin  Amplitude=80  Frequency=2*pi*0.005
  Sine Wave1 : Sin  Amplitude=80  Frequency=2*pi*0.005  Phase=pi/2
  Slider1 : SliderBlock  ScaleMin=-20  ScaleMax=20
  Slider2 : SliderBlock  ScaleMin=-180  ScaleMax=180
  Slider3 : SliderBlock
  Slider4 : SliderBlock  ScaleMin=-20  ScaleMax=20
  Terminator : Terminator
  desX : Constant  Value=0  SampleTime=-1
  desY : Constant  Value=0  SampleTime=-1
  des_alt : Constant  Value=8  SampleTime=-1
  des_yaw : Constant  Value=0  SampleTime=-1
  Desired Position : Outport
  wires:
  des_alt/1 -> Gain/1
  desY/1 -> Manual Switch1/1
  Sine Wave/1 -> Manual Switch/2
  desX/1 -> Manual Switch/1
  Manual Switch1/1 -> Mux/2  "des_y"
  des_yaw/1 -> Degrees to Radians/1
  Manual Switch/1 -> Mux/1  "des_x"
  Sine Wave1/1 -> Manual Switch1/2
  Mux/1 -> Desired Position/1
  Current Position/1 -> Terminator/1
  Gain/1 -> Mux/3
  Degrees to Radians/1 -> Mux/4

== system HITL_HEXA_MISSION/Navigation/Quadcopter Navigation Algorithm/Path Correction from Onboard Computer ==
  Current Position : Inport
  Bus Selector : BusSelector  OutputSignals=position,yaw
  Bus Selector1 : BusSelector  OutputSignals=waypoints
  Cast : DataTypeConversion  SaturateOnIntegerOverflow=off  RndMeth=Floor
  Cast1 : DataTypeConversion  SaturateOnIntegerOverflow=off  RndMeth=Floor
  "Define WP Yaw Values " : Subsystem
  Guidance Subsystem : Subsystem
      settings: PortSchema="{\"entries\":[{\"content\":{\"sides\":[{\"content\":{\"connectorIds\":[\"In1\",\"In2\",\"In3\",\"In4\",\"In5\",\"In6\",\"In7\"]},\"type\":\"ConnectorPlacement.EquallySpacedRectSide\",\"uuid\":\"e9e96be5-af21-4911-860e-f3d41d3d51a5\"},{\"content\":{\"connectorIds\":[\"Out1\"],\"side\":\"RIGHT\"},\"type\":\"ConnectorPlacement.EquallySpacedRectSide\",\"uuid\":\"1d190cc4-2348-4eca-a529-c9f1d728b718\"},{\"content\":{\"connectorIds\":[\"In8\"],\"side\":\"TOP\"},\"type\":\"ConnectorPlacement.EquallySpacedRectSide\",\"uuid\":\"c248d3d5-3b30-416c-a277-519f6ee966ff\"},{\"content\":{\"connectorIds\":[\"In9\",\"In10\"],\"side\":\"BOTTOM\"},\"type\":\"ConnectorPlacement.EquallySpacedRectSide\",\"uuid\":\"2b8da87f-17bd-449d-af9e-128c1548c7b5\"}]},\"type\":\"ConnectorPlacement.EquallySpacedConnector\",\"uuid\":\"bbf0c511-85fc-440a-b356-10e645af4727\"}],\"packageUris\":[\"http://schema.mathworks.com/mf0/Connector/R2020b\"],\"version\":\"1.0\"}"
  NaN Check : Subsystem
  NaN Check1 : Subsystem
  NaN Check2 : Subsystem
  NaN Check3 : Subsystem
  NaN Check4 : Subsystem
  NaN Check5 : Subsystem
  PX4 uORB Read : px4uORBlib/PX4 uORB Read  uORBTopic=vehicle_trajectory_waypoint  selectInstance=vehicle_trajectory_waypoint_desired  SampleTime=SampleTime  BlockingMode=off  BlockTimeout=1e-3
  Read Position Setpoint from Mission set in QGC : px4lib/PX4 Read Position Setpoint  coordinateFrame=Local Coordinates (NED)  SampleTime=SampleTime  positionSetpointBus=on  trajectoryWaypointsBus=on  onboardFailsafeFlag=off  onboardEnableStatus=on
  Selector : Selector  InputPortWidth=5  IndexOptions=Index vector (dialog)  Indices=2  OutputSizes=1
  Terminator : Terminator
  Terminator1 : Terminator
  Desired Position : Outport
  wires:
  Read Position Setpoint from Mission set in QGC/2 -> NaN Check1/1(In1)  "Current"
  Read Position Setpoint from Mission set in QGC/4 -> Guidance Subsystem/4(Waypoint Type)
  Read Position Setpoint from Mission set in QGC/1 -> NaN Check/1(In1)  "Previous"
  Guidance Subsystem/1(Desired_Pose) -> Desired Position/1
  Read Position Setpoint from Mission set in QGC/3 -> NaN Check2/1(In1)  "Next"
  Current Position/1 -> Guidance Subsystem/8(Current Position)
  Read Position Setpoint from Mission set in QGC/7 -> Terminator/1
  Read Position Setpoint from Mission set in QGC/6 -> "Define WP Yaw Values "/2(Trajectory Waypoint)
  Read Position Setpoint from Mission set in QGC/5 -> "Define WP Yaw Values "/1(position setpoint)
  "Define WP Yaw Values "/3(Next WP Yaw) -> NaN Check5/1(In1)
  "Define WP Yaw Values "/2(Current WP Yaw) -> NaN Check4/1(In1)
  "Define WP Yaw Values "/1(Previous WP Yaw) -> NaN Check3/1(In1)
  PX4 uORB Read/1 -> Terminator1/1
  Bus Selector/1 -> Cast/1  "<position>"
  PX4 uORB Read/2 -> Bus Selector1/1
  Selector/1 -> Bus Selector/1
  Bus Selector/2 -> Cast1/1  "<yaw>"
  Bus Selector1/1 -> Selector/1  "<waypoints>"
  Cast/1 -> Guidance Subsystem/9(Planned_current_pos)
  Cast1/1 -> Guidance Subsystem/10(planned_current_yaw)
  NaN Check/1(Out1) -> Guidance Subsystem/1(Previous WP)
  NaN Check1/1(Out1) -> Guidance Subsystem/2(Current WP)
  NaN Check2/1(Out1) -> Guidance Subsystem/3(Next WP)
  NaN Check3/1(Out1) -> Guidance Subsystem/5(Previous WP Yaw)
  NaN Check4/1(Out1) -> Guidance Subsystem/6(Current WP Yaw)
  NaN Check5/1(Out1) -> Guidance Subsystem/7(Next WP Yaw)

== system HITL_HEXA_MISSION/Navigation/Quadcopter Navigation Algorithm/Read waypoint from QGroundControl Mission ==
  Current Position : Inport
  Guidance Subsystem : Subsystem
      settings: PortSchema="{\"entries\":[{\"content\":{\"sides\":[{\"content\":{\"connectorIds\":[\"In1\",\"In2\",\"In3\",\"In4\"]},\"type\":\"ConnectorPlacement.EquallySpacedRectSide\",\"uuid\":\"e9e96be5-af21-4911-860e-f3d41d3d51a5\"},{\"content\":{\"connectorIds\":[\"Out1\"],\"side\":\"RIGHT\"},\"type\":\"ConnectorPlacement.EquallySpacedRectSide\",\"uuid\":\"1d190cc4-2348-4eca-a529-c9f1d728b718\"},{\"content\":{\"connectorIds\":[\"In5\"],\"side\":\"TOP\"},\"type\":\"ConnectorPlacement.EquallySpacedRectSide\",\"uuid\":\"c248d3d5-3b30-416c-a277-519f6ee966ff\"}]},\"type\":\"ConnectorPlacement.EquallySpacedConnector\",\"uuid\":\"bbf0c511-85fc-440a-b356-10e645af4727\"}],\"packageUris\":[\"http://schema.mathworks.com/mf0/Connector/R2020b\"],\"version\":\"1.0\"}"
  Read Position Setpoint from Mission set in QGC : px4lib/PX4 Read Position Setpoint  coordinateFrame=Local Coordinates (NED)  SampleTime=-1  positionSetpointBus=off  trajectoryWaypointsBus=off  onboardFailsafeFlag=off  onboardEnableStatus=off
  Desired Position : Outport
  wires:
  Read Position Setpoint from Mission set in QGC/1 -> Guidance Subsystem/1(Previous WP)  "Previous"
  Read Position Setpoint from Mission set in QGC/4 -> Guidance Subsystem/4(Waypoint Type)
  Read Position Setpoint from Mission set in QGC/2 -> Guidance Subsystem/2(Current WP)  "Current"
  Guidance Subsystem/1(Desired_Pose) -> Desired Position/1
  Read Position Setpoint from Mission set in QGC/3 -> Guidance Subsystem/3(Next WP)  "Next"
  Current Position/1 -> Guidance Subsystem/5(Current Position)

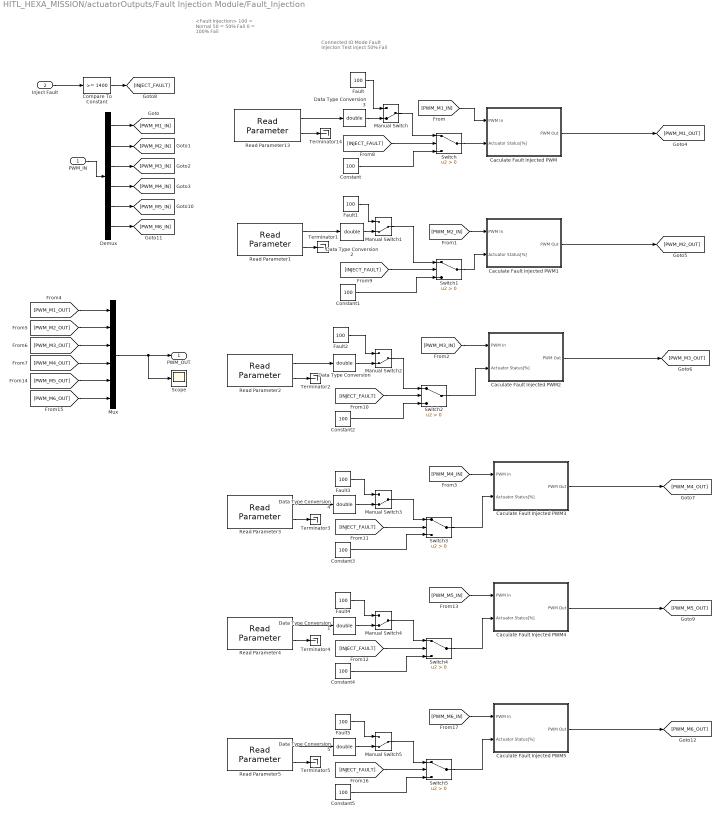
== system HITL_HEXA_MISSION/actuatorOutputs/Fault Injection Module/Fault_Injection ==
  note: Connected IO Mode
      | Fault Injecton Test
      |
      | inject 50% Fail
  note: <Fault Injection>
      | 100 = Nornal
      | 50 = 50% Fail
      | 0 = 100% Fail
  PWM_IN : Inport
  Inject Fault : Inport  Port=2
  Caculate Fault Injected PWM : Subsystem
  Caculate Fault Injected PWM1 : Subsystem
  Caculate Fault Injected PWM2 : Subsystem
  Caculate Fault Injected PWM3 : Subsystem
  Caculate Fault Injected PWM4 : Subsystem
  Caculate Fault Injected PWM5 : Subsystem
  Compare To Constant : simulink/Logic and Bit Operations/Compare To Constant  relop=>=  const=1400  OutDataTypeStr=boolean
  Constant{,1..5} (6 alike) : Constant  Value=100
  Data Type Conversion{,1..5} (6 alike) : DataTypeConversion  OutDataTypeStr=double  SaturateOnIntegerOverflow=off  RndMeth=Floor
  Demux : Demux  Outputs=6
  Fault{,1..5} (6 alike) : Constant  Value=100
  Manual Switch{,1..5} (6 alike) : ManualSwitch  CurrentSetting=0
  Mux : Mux  Inputs=6
  Read Parameter1 : px4lib/Read Parameter  ParameterName=FDD_M2_STATUS  DataType=INT32  SampleTime=-1
  Read Parameter13 : px4lib/Read Parameter  ParameterName=FDD_M1_STATUS  DataType=INT32  SampleTime=-1
  Read Parameter2 : px4lib/Read Parameter  ParameterName=FDD_M3_STATUS  DataType=INT32  SampleTime=-1
  Read Parameter3 : px4lib/Read Parameter  ParameterName=FDD_M4_STATUS  DataType=INT32  SampleTime=-1
  Read Parameter4 : px4lib/Read Parameter  ParameterName=FDD_M5_STATUS  DataType=INT32  SampleTime=-1
  Read Parameter5 : px4lib/Read Parameter  ParameterName=FDD_M6_STATUS  DataType=INT32  SampleTime=-1
  Scope : Scope
  Switch{,1..5} (6 alike) : Switch  Criteria=u2 > Threshold  SaturateOnIntegerOverflow=off  InputSameDT=off
  Terminator{1..5,14} (6 alike) : Terminator
  PWM_OUT : Outport
  wires:
  Read Parameter13/2 -> Terminator14/1
  Read Parameter1/2 -> Terminator1/1
  Read Parameter2/2 -> Terminator2/1
  Read Parameter2/1 -> Data Type Conversion/1
  Read Parameter3/2 -> Terminator3/1
  Read Parameter3/1 -> Data Type Conversion4/1
  Data Type Conversion/1 -> Manual Switch2/2
  Data Type Conversion4/1 -> Manual Switch3/2
  Read Parameter13/1 -> Data Type Conversion3/1
  Read Parameter1/1 -> Data Type Conversion2/1
  Data Type Conversion3/1 -> Manual Switch/2
  Fault/1 -> Manual Switch/1
  Data Type Conversion2/1 -> Manual Switch1/2
  Fault1/1 -> Manual Switch1/1
  Fault2/1 -> Manual Switch2/1
  Fault3/1 -> Manual Switch3/1
  PWM_IN/1 -> Demux/1
  Demux/1 -> [PWM_M1_IN]
  Demux/2 -> [PWM_M2_IN]
  Demux/3 -> [PWM_M3_IN]
  Demux/4 -> [PWM_M4_IN]
  [PWM_M1_IN] -> Caculate Fault Injected PWM/1(PWM In)
  [PWM_M2_IN] -> Caculate Fault Injected PWM1/1(PWM In)
  [PWM_M3_IN] -> Caculate Fault Injected PWM2/1(PWM In)
  [PWM_M4_IN] -> Caculate Fault Injected PWM3/1(PWM In)
  Mux/1 -> Scope/1, PWM_OUT/1
  [PWM_M1_OUT] -> Mux/1
  [PWM_M2_OUT] -> Mux/2
  [PWM_M3_OUT] -> Mux/3
  [PWM_M4_OUT] -> Mux/4
  Inject Fault/1 -> Compare To Constant/1
  Compare To Constant/1 -> [INJECT_FAULT]
  Manual Switch/1 -> Switch/1
  Switch/1 -> Caculate Fault Injected PWM/2(" Actuator Status[%]")
  [INJECT_FAULT] -> Switch/2
  Constant/1 -> Switch/3
  Constant1/1 -> Switch1/3
  [INJECT_FAULT] -> Switch1/2
  Switch1/1 -> Caculate Fault Injected PWM1/2(" Actuator Status[%]")
  Manual Switch1/1 -> Switch1/1
  Switch2/1 -> Caculate Fault Injected PWM2/2(" Actuator Status[%]")
  Constant2/1 -> Switch2/3
  [INJECT_FAULT] -> Switch2/2
  Manual Switch2/1 -> Switch2/1
  Switch3/1 -> Caculate Fault Injected PWM3/2(" Actuator Status[%]")
  Constant3/1 -> Switch3/3
  [INJECT_FAULT] -> Switch3/2
  Manual Switch3/1 -> Switch3/1
  [PWM_M5_IN] -> Caculate Fault Injected PWM4/1(PWM In)
  Read Parameter4/1 -> Data Type Conversion1/1
  Fault4/1 -> Manual Switch4/1
  Switch4/1 -> Caculate Fault Injected PWM4/2(" Actuator Status[%]")
  Manual Switch4/1 -> Switch4/1
  Constant4/1 -> Switch4/3
  Data Type Conversion1/1 -> Manual Switch4/2
  Read Parameter4/2 -> Terminator4/1
  [INJECT_FAULT] -> Switch4/2
  Demux/5 -> [PWM_M5_IN]
  Demux/6 -> [PWM_M6_IN]
  [PWM_M5_OUT] -> Mux/5
  [PWM_M6_OUT] -> Mux/6
  Fault5/1 -> Manual Switch5/1
  [PWM_M6_IN] -> Caculate Fault Injected PWM5/1(PWM In)
  Manual Switch5/1 -> Switch5/1
  Read Parameter5/2 -> Terminator5/1
  [INJECT_FAULT] -> Switch5/2
  Read Parameter5/1 -> Data Type Conversion5/1
  Constant5/1 -> Switch5/3
  Data Type Conversion5/1 -> Manual Switch5/2
  Switch5/1 -> Caculate Fault Injected PWM5/2(" Actuator Status[%]")
  Caculate Fault Injected PWM/1(PWM Out) -> [PWM_M1_OUT]
  Caculate Fault Injected PWM1/1(PWM Out) -> [PWM_M2_OUT]
  Caculate Fault Injected PWM2/1(PWM Out) -> [PWM_M3_OUT]
  Caculate Fault Injected PWM3/1(PWM Out) -> [PWM_M4_OUT]
  Caculate Fault Injected PWM4/1(PWM Out) -> [PWM_M5_OUT]
  Caculate Fault Injected PWM5/1(PWM Out) -> [PWM_M6_OUT]

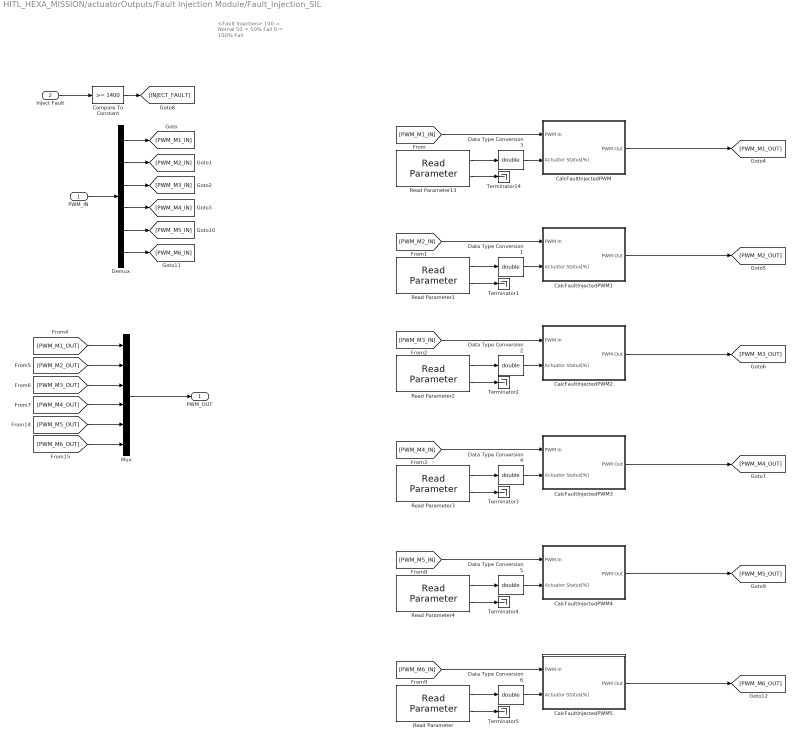
== system HITL_HEXA_MISSION/actuatorOutputs/Fault Injection Module/Fault_Injection_SIL ==
  note: <Fault Injection>
      | 100 = Nornal
      | 50 = 50% Fail
      | 0 = 100% Fail
  PWM_IN : Inport
  Inject Fault : Inport  Port=2
  CalcFaultInjectedPWM : Subsystem  TreatAsAtomicUnit=on  RTWFcnName=calcFaultInjectedPWM  RTWFileName=calcFaultInjectedPWM
      settings: RTWFcnNameOpts=User specified  RTWFileNameOpts=User specified
  CalcFaultInjectedPWM1 : Subsystem  TreatAsAtomicUnit=on  RTWFcnName=calcFaultInjectedPWM  RTWFileName=calcFaultInjectedPWM
      settings: RTWFcnNameOpts=User specified  RTWFileNameOpts=User specified
  CalcFaultInjectedPWM2 : Subsystem  TreatAsAtomicUnit=on  RTWFcnName=calcFaultInjectedPWM  RTWFileName=calcFaultInjectedPWM
      settings: RTWFcnNameOpts=User specified  RTWFileNameOpts=User specified
  CalcFaultInjectedPWM3 : Subsystem  TreatAsAtomicUnit=on  RTWFcnName=calcFaultInjectedPWM  RTWFileName=calcFaultInjectedPWM
      settings: RTWFcnNameOpts=User specified  RTWFileNameOpts=User specified
  CalcFaultInjectedPWM4 : Subsystem  TreatAsAtomicUnit=on  RTWFcnName=calcFaultInjectedPWM  RTWFileName=calcFaultInjectedPWM
      settings: RTWFcnNameOpts=User specified  RTWFileNameOpts=User specified
  CalcFaultInjectedPWM5 : Subsystem  TreatAsAtomicUnit=on  RTWFcnName=calcFaultInjectedPWM  RTWFileName=calcFaultInjectedPWM
      settings: RTWFcnNameOpts=User specified  RTWFileNameOpts=User specified
  Compare To Constant : simulink/Logic and Bit Operations/Compare To Constant  relop=>=  const=1400  OutDataTypeStr=boolean
  Data Type Conversion{1..6} (6 alike) : DataTypeConversion  OutDataTypeStr=double  SaturateOnIntegerOverflow=off  RndMeth=Floor
  Demux : Demux  Outputs=6
  Mux : Mux  Inputs=6
  Read Parameter : px4lib/Read Parameter  ParameterName=FDD_M6_STATUS  DataType=FLOAT  SampleTime=-1
  Read Parameter1 : px4lib/Read Parameter  ParameterName=FDD_M2_STATUS  DataType=INT32  SampleTime=-1
  Read Parameter13 : px4lib/Read Parameter  ParameterName=FDD_M1_STATUS  DataType=INT32  SampleTime=-1
  Read Parameter2 : px4lib/Read Parameter  ParameterName=FDD_M3_STATUS  DataType=INT32  SampleTime=-1
  Read Parameter3 : px4lib/Read Parameter  ParameterName=FDD_M4_STATUS  DataType=INT32  SampleTime=-1
  Read Parameter4 : px4lib/Read Parameter  ParameterName=FDD_M5_STATUS  DataType=INT32  SampleTime=-1
  Terminator{1..5,14} (6 alike) : Terminator
  PWM_OUT : Outport
  wires:
  Read Parameter13/2 -> Terminator14/1
  Read Parameter13/1 -> Data Type Conversion3/1
  PWM_IN/1 -> Demux/1
  Demux/1 -> [PWM_M1_IN]
  Demux/2 -> [PWM_M2_IN]
  Demux/3 -> [PWM_M3_IN]
  Demux/4 -> [PWM_M4_IN]
  [PWM_M1_IN] -> CalcFaultInjectedPWM/1(PWM In)
  Mux/1 -> PWM_OUT/1
  [PWM_M1_OUT] -> Mux/1
  [PWM_M2_OUT] -> Mux/2
  [PWM_M3_OUT] -> Mux/3
  [PWM_M4_OUT] -> Mux/4
  Inject Fault/1 -> Compare To Constant/1
  Compare To Constant/1 -> [INJECT_FAULT]
  Demux/5 -> [PWM_M5_IN]
  Demux/6 -> [PWM_M6_IN]
  [PWM_M5_OUT] -> Mux/5
  [PWM_M6_OUT] -> Mux/6
  CalcFaultInjectedPWM/1(PWM Out) -> [PWM_M1_OUT]
  Data Type Conversion3/1 -> CalcFaultInjectedPWM/2(" Actuator Status[%]")
  Read Parameter1/2 -> Terminator1/1
  CalcFaultInjectedPWM1/1(PWM Out) -> [PWM_M2_OUT]
  Read Parameter1/1 -> Data Type Conversion1/1
  [PWM_M2_IN] -> CalcFaultInjectedPWM1/1(PWM In)
  Data Type Conversion1/1 -> CalcFaultInjectedPWM1/2(" Actuator Status[%]")
  Read Parameter2/2 -> Terminator2/1
  CalcFaultInjectedPWM2/1(PWM Out) -> [PWM_M3_OUT]
  Read Parameter2/1 -> Data Type Conversion2/1
  [PWM_M3_IN] -> CalcFaultInjectedPWM2/1(PWM In)
  Data Type Conversion2/1 -> CalcFaultInjectedPWM2/2(" Actuator Status[%]")
  Read Parameter3/2 -> Terminator3/1
  CalcFaultInjectedPWM3/1(PWM Out) -> [PWM_M4_OUT]
  Read Parameter3/1 -> Data Type Conversion4/1
  [PWM_M4_IN] -> CalcFaultInjectedPWM3/1(PWM In)
  Data Type Conversion4/1 -> CalcFaultInjectedPWM3/2(" Actuator Status[%]")
  Read Parameter4/2 -> Terminator4/1
  CalcFaultInjectedPWM4/1(PWM Out) -> [PWM_M5_OUT]
  Read Parameter4/1 -> Data Type Conversion5/1
  [PWM_M5_IN] -> CalcFaultInjectedPWM4/1(PWM In)
  Data Type Conversion5/1 -> CalcFaultInjectedPWM4/2(" Actuator Status[%]")
  Read Parameter/2 -> Terminator5/1
  CalcFaultInjectedPWM5/1(PWM Out) -> [PWM_M6_OUT]
  Read Parameter/1 -> Data Type Conversion6/1
  [PWM_M6_IN] -> CalcFaultInjectedPWM5/1(PWM In)
  Data Type Conversion6/1 -> CalcFaultInjectedPWM5/2(" Actuator Status[%]")

== system HITL_HEXA_MISSION/Actuator/Custom Mixer and PWM Output Block/Fault_Injection/Caculate Fault Injected PWM ==
  note: $\text{Fault Injection Formula} \\ NormalPWM = x, ActuatorStatus = e \\ {(x-1100)\times{e} \over{100}} + 1100$
  PWM In : Inport
  " Actuator Status[%]" : Inport  Port=2
  Add : Sum  Inputs=-+
  Constant : Constant  Value=1100
  Gain : Gain  Gain=0.01
  IDLE PWM : Constant  Value=1100
  Product : Product
  Saturation1 : Saturate  UpperLimit=1  LowerLimit=0
  Sum : Sum  Inputs=|++
  PWM Out : Outport
  wires:
  Gain/1 -> Saturation1/1
  Product/1 -> Sum/1
  Constant/1 -> Sum/2
  Add/1 -> Product/1
  Saturation1/1 -> Product/2
  IDLE PWM/1 -> Add/1
  Sum/1 -> PWM Out/1
  PWM In/1 -> Add/2
  " Actuator Status[%]"/1 -> Gain/1
